simulink model "modelo_ARX"  (R2015a)
settings: Solver=ode45  StartTime=0.0  StopTime=200  RelTol=1e-3
values from neighbouring files (symbols this model uses):
  lambda = 1    [generar_prbs.m]    (also in parametros_ident.m = 0.995)
undefined symbols (not defined in the file or in its folder): sigbuilder_block
settings Model: Creator=u_labelectro  LastModifiedBy=Luis
settings DebuggingCC: UnderspecifiedInitializationDetection=Classic  MergeDetectMultiDrivingBlocksExec=none  SolverPrmCheckMsg=warning  StateNameClashWarn=warning

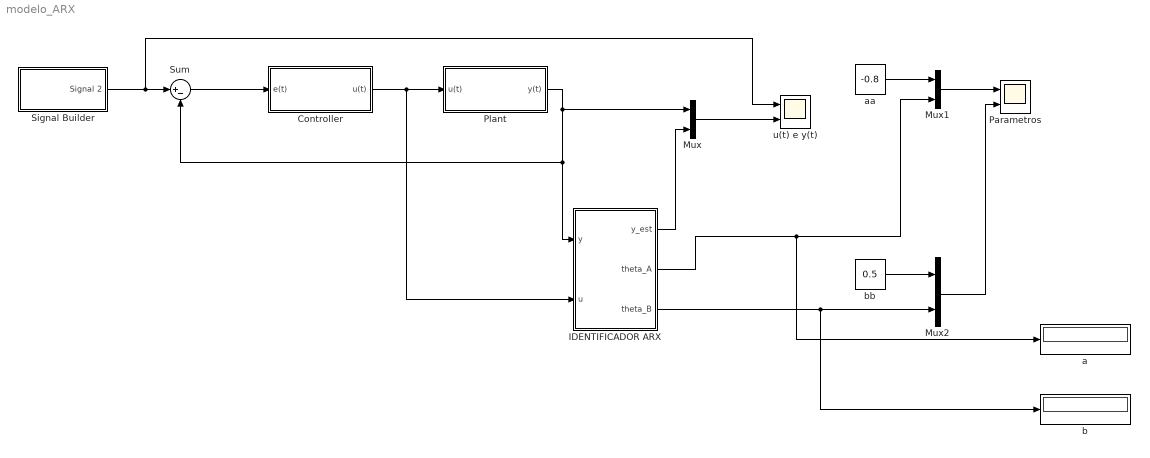
== system modelo_ARX ==
  Controller : Subsystem
  IDENTIFICADOR ARX : Subsystem
  Mux : Mux  Inputs=2
  Mux1 : Mux  Inputs=2
  Mux2 : Mux  Inputs=2
  Parametros : Scope  NumInputPorts=2
      settings: YMin=-5~-5  YMax=5~5
  Plant : Subsystem
  Signal Builder : Subsystem  Tag=STV Subsys  LoadFcn=sigbuilder_block('load',[6 28.5 1068 583.5 ]);  StartFcn=sigbuilder_block('start');  StopFcn=sigbuilder_block('stop');  ClipboardFcn=sigbuilder_block('clipboard');  mask(Sigbuilder block){}
      mask help: Simulink:masks:SigbuilderBlock_MD
      mask init:
      | if ~strcmp(get_param(bdroot(gcbh),'SimulationStatus'),'stopped') tuvar = sigbuilder_block('maskInit'); end
      settings: CopyFcn=sigbuilder_block('copy');  DeleteFcn=sigbuilder_block('delete');  ModelCloseFcn=sigbuilder_block('modelClose');  PreSaveFcn=sigbuilder_block('preSave');  PauseFcn=sigbuilder_block('pause');  ContinueFcn=sigbuilder_block('continue');  NameChangeFcn=sigbuilder_block('namechange');  OpenFcn=sigbuilder_block('open',[6 28.5 1068 583.5 ]);  CloseFcn=sigbuilder_block('close');
      mask Display: plot(0, 0, 100, 100,[2, 2, 32, 32, 2], [68, 8, 8, 68, 68],[32, 2], [38, 38], [32, 19, 2],[53, 60, 44], [32, 17, 17, 2],[16, 16, 31, 31]);txt = getActiveGroup(gcbh);text(2, 100, txt,'verticalAlignment', 'top');
  Sum : Sum  Inputs=|+-
  a : Display
  aa : Constant  Value=-0.8
  b : Display
  bb : Constant  Value=0.5
  u(t) e y(t) : Scope  NumInputPorts=2
      settings: YMin=-5~-5  YMax=5~5  SaveName=ScopeData2
  wires:
  Signal Builder/1(Signal 2) -> u(t) e y(t)/1, Sum/1
  Sum/1 -> Controller/1(e(t))
  Controller/1(u(t)) -> IDENTIFICADOR ARX/2(u), Plant/1(u(t))
  Plant/1(y(t)) -> Mux/1, Sum/2, IDENTIFICADOR ARX/1(y)
  IDENTIFICADOR ARX/1(y_est) -> Mux/2
  Mux/1 -> u(t) e y(t)/2
  aa/1 -> Mux1/1
  IDENTIFICADOR ARX/2(theta_A) -> a/1, Mux1/2
  bb/1 -> Mux2/1
  IDENTIFICADOR ARX/3(theta_B) -> b/1, Mux2/2
  Mux1/1 -> Parametros/1
  Mux2/1 -> Parametros/2

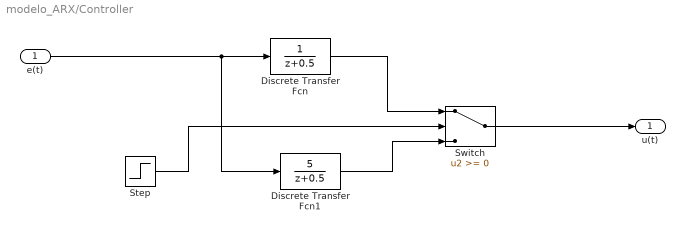
== system modelo_ARX/Controller ==
  e(t) : Inport
  Discrete Transfer Fcn : DiscreteTransferFcn  SampleTime=0.01
  Discrete Transfer Fcn1 : DiscreteTransferFcn  Numerator=[5]  SampleTime=0.01
  Step : Step  Time=50  SampleTime=0
  Switch : Switch
  u(t) : Outport
  wires:
  Step/1 -> Switch/2
  Discrete Transfer Fcn1/1 -> Switch/3
  Discrete Transfer Fcn/1 -> Switch/1
  e(t)/1 -> Discrete Transfer Fcn1/1, Discrete Transfer Fcn/1
  Switch/1 -> u(t)/1

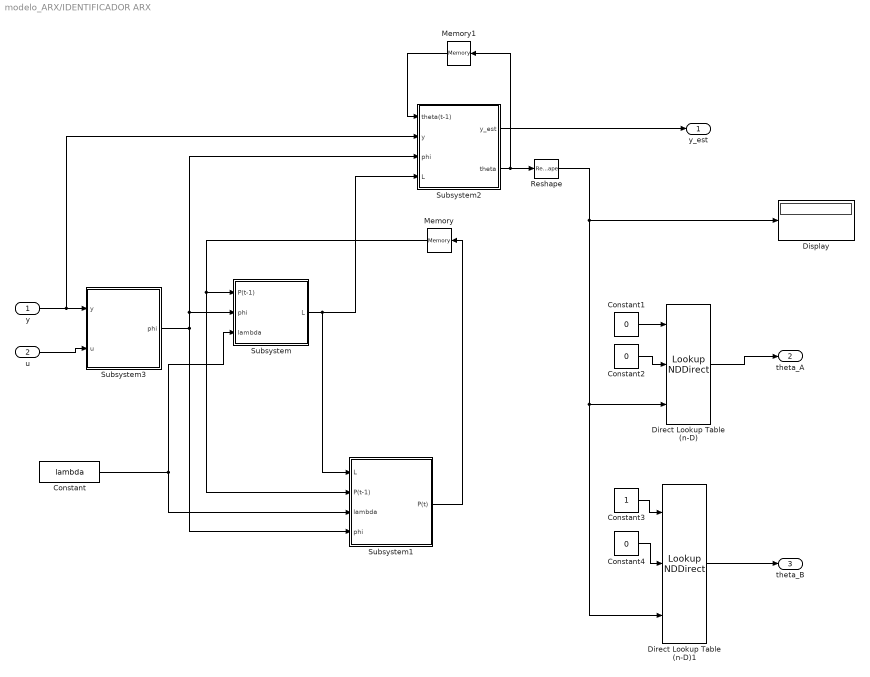
== system modelo_ARX/IDENTIFICADOR ARX ==
  y : Inport
  u : Inport  Port=2
  Constant : Constant  Value=lambda
  Constant1 : Constant  Value=0
  Constant2 : Constant  Value=0
  Constant3 : Constant
  Constant4 : Constant  Value=0
  Direct Lookup Table (n-D) : LookupNDDirect  TableIsInput=on  Table=[4 5 ;16 19 ]  DiagnosticForOutOfRangeInput=Error
  Direct Lookup Table (n-D)1 : LookupNDDirect  TableIsInput=on  Table=[4 5 ;16 19 ]  DiagnosticForOutOfRangeInput=Error
  Display : Display
  Memory : Memory  X0=1e6*eye(2)
  Memory1 : Memory
  Reshape : Reshape  OutputDimensionality=Column vector (2-D)
  Subsystem : Subsystem
  Subsystem1 : Subsystem
  Subsystem2 : Subsystem
  Subsystem3 : Subsystem
  y_est : Outport
  theta_A : Outport  Port=2
  theta_B : Outport  Port=3
  wires:
  y/1 -> Subsystem2/2(y), Subsystem3/1(y)
  Subsystem3/1(phi) -> Subsystem1/4(phi), Subsystem2/3(phi), Subsystem/2(phi)
  Subsystem/1(L) -> Subsystem1/1(L), Subsystem2/4(L)
  u/1 -> Subsystem3/2(u)
  Constant/1 -> Subsystem1/3(lambda), Subsystem/3(lambda)
  Subsystem1/1(P(t)) -> Memory/1
  Memory/1 -> Subsystem1/2(P(t-1)), Subsystem/1(P(t-1))
  Subsystem2/1(y_est) -> y_est/1
  Subsystem2/2(theta) -> Reshape/1, Memory1/1
  Memory1/1 -> Subsystem2/1(theta(t-1))
  Constant4/1 -> Direct Lookup Table (n-D)1/2
  Constant3/1 -> Direct Lookup Table (n-D)1/1
  Constant2/1 -> Direct Lookup Table (n-D)/2
  Constant1/1 -> Direct Lookup Table (n-D)/1
  Reshape/1 -> Direct Lookup Table (n-D)1/3, Direct Lookup Table (n-D)/3, Display/1
  Direct Lookup Table (n-D)/1 -> theta_A/1
  Direct Lookup Table (n-D)1/1 -> theta_B/1

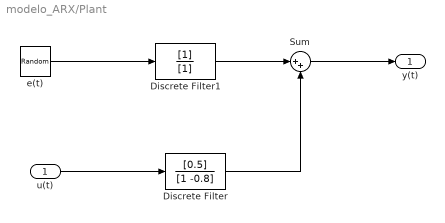
== system modelo_ARX/Plant ==
  u(t) : Inport
  Discrete Filter : DiscreteFilter  Numerator=[0.5]  Denominator=[1 -0.8]  SampleTime=0.01
  Discrete Filter1 : DiscreteFilter  Denominator=[1]
  Sum : Sum  Inputs=|++
  e(t) : RandomNumber  Variance=0.001  SampleTime=0.1
  y(t) : Outport
  wires:
  Discrete Filter/1 -> Sum/2
  Discrete Filter1/1 -> Sum/1
  Sum/1 -> y(t)/1
  u(t)/1 -> Discrete Filter/1
  e(t)/1 -> Discrete Filter1/1

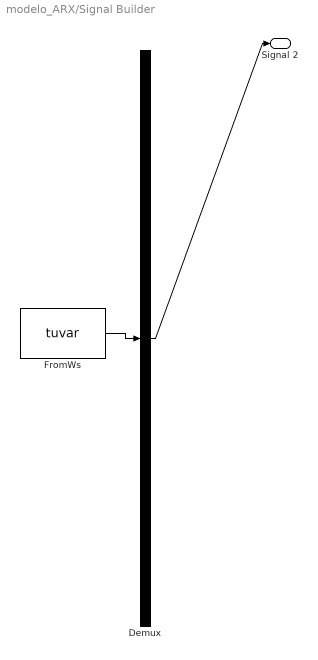
== system modelo_ARX/Signal Builder ==
  Demux : Demux  Tag=STV Demux  Outputs=1
  FromWs : FromWorkspace  Tag=STV FromWs  VariableName=tuvar  SampleTime=0
      SigBuilderData=|
      | common.afterFinalStr = 'Extrapolate'
      | common.sampleTime = 0
      | dataSet.timeRange = [0 100]
      | dataSet.name = 'Group 1'
      | sbobj.Groups.Name = 'Group 1'
      | sbobj.Groups.Signals.Name = 'Signal 2'
      | sbobj.Groups.Signals.XData = [0 10 10 20 100]
      | sbobj.Groups.Signals.YData = [0 0.002 0.496 0.5 0.5]
      | sbobj.Groups.TimeRange = [0 100]
  Signal 2 : Outport  Tag=STV Outport
  wires:
  FromWs/1 -> Demux/1
  Demux/1 -> Signal 2/1

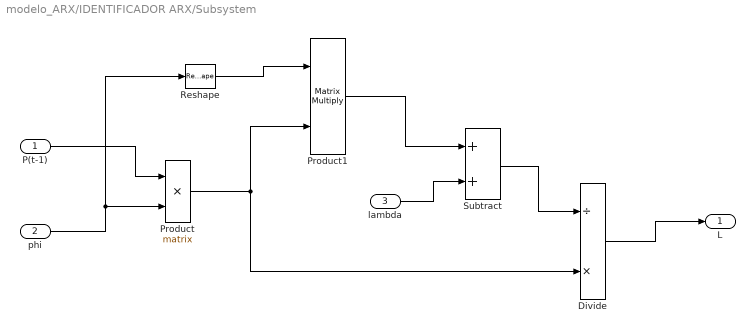
== system modelo_ARX/IDENTIFICADOR ARX/Subsystem ==
  P(t-1) : Inport
  phi : Inport  Port=2
  lambda : Inport  Port=3
  Divide : Product  Inputs=/*
  Product : Product  Multiplication=Matrix(*)
  Product1 : Product  Multiplication=Matrix(*)
  Reshape : Reshape  OutputDimensionality=Row vector (2-D)
  Subtract : Sum
  L : Outport
  wires:
  Divide/1 -> L/1
  Subtract/1 -> Divide/1
  phi/1 -> Reshape/1, Product/2
  Reshape/1 -> Product1/1
  Product1/1 -> Subtract/1
  lambda/1 -> Subtract/2
  Product/1 -> Product1/2, Divide/2
  P(t-1)/1 -> Product/1

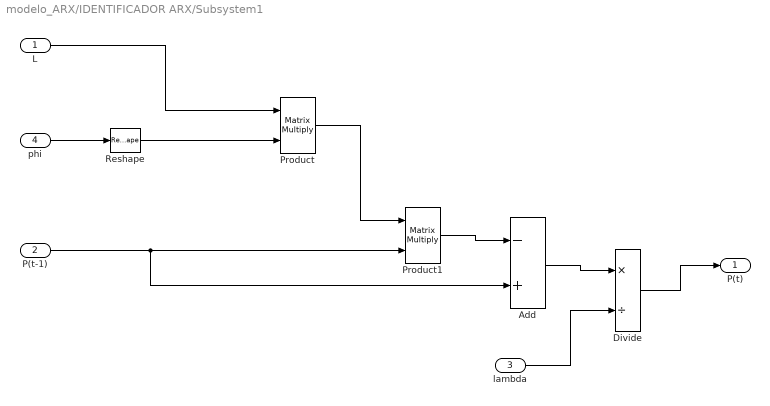
== system modelo_ARX/IDENTIFICADOR ARX/Subsystem1 ==
  L : Inport
  P(t-1) : Inport  Port=2
  lambda : Inport  Port=3
  phi : Inport  Port=4
  Add : Sum  Inputs=-+
  Divide : Product  Inputs=*/
  Product : Product  Multiplication=Matrix(*)
  Product1 : Product  Multiplication=Matrix(*)
  Reshape : Reshape  OutputDimensionality=Row vector (2-D)
  P(t) : Outport
  wires:
  L/1 -> Product/1
  phi/1 -> Reshape/1
  Reshape/1 -> Product/2
  Product/1 -> Product1/1
  P(t-1)/1 -> Add/2, Product1/2
  Product1/1 -> Add/1
  Add/1 -> Divide/1
  Divide/1 -> P(t)/1
  lambda/1 -> Divide/2

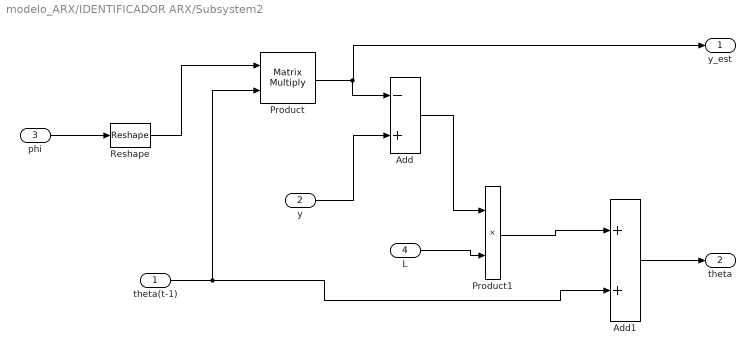
== system modelo_ARX/IDENTIFICADOR ARX/Subsystem2 ==
  theta(t-1) : Inport
  y : Inport  Port=2
  phi : Inport  Port=3
  L : Inport  Port=4
  Add : Sum  Inputs=-+
  Add1 : Sum
  Product : Product  Multiplication=Matrix(*)
  Product1 : Product
  Reshape : Reshape  OutputDimensionality=Row vector (2-D)
  y_est : Outport
  theta : Outport  Port=2
  wires:
  Product/1 -> Add/1, y_est/1
  y/1 -> Add/2
  L/1 -> Product1/2
  Add/1 -> Product1/1
  Product1/1 -> Add1/1
  Add1/1 -> theta/1
  theta(t-1)/1 -> Product/2, Add1/2
  Reshape/1 -> Product/1
  phi/1 -> Reshape/1

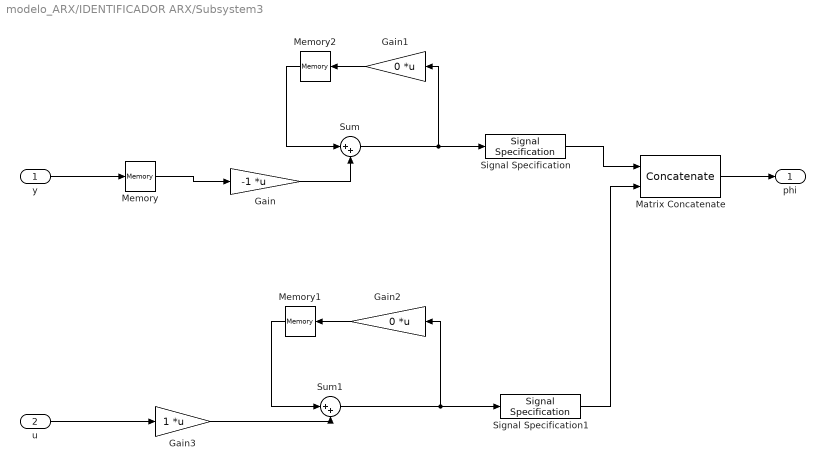
== system modelo_ARX/IDENTIFICADOR ARX/Subsystem3 ==
  y : Inport
  u : Inport  Port=2
  Gain : Gain  Gain=-1  Multiplication=Matrix(K*u)
  Gain1 : Gain  Gain=0  Multiplication=Matrix(K*u)
  Gain2 : Gain  Gain=0  Multiplication=Matrix(K*u)
  Gain3 : Gain  Multiplication=Matrix(K*u)
  Matrix Concatenate : Concatenate  Mode=Multidimensional array
  Memory : Memory
  Memory1 : Memory
  Memory2 : Memory
  Signal Specification : SignalSpecification  Dimensions=[1 1]
  Signal Specification1 : SignalSpecification  Dimensions=[1 1]
  Sum : Sum  Inputs=|++
  Sum1 : Sum  Inputs=|++
  phi : Outport
  wires:
  Sum/1 -> Gain1/1, Signal Specification/1
  Gain1/1 -> Memory2/1
  Memory2/1 -> Sum/1
  Gain/1 -> Sum/2
  Memory/1 -> Gain/1
  y/1 -> Memory/1
  Gain2/1 -> Memory1/1
  u/1 -> Gain3/1
  Gain3/1 -> Sum1/2
  Memory1/1 -> Sum1/1
  Sum1/1 -> Signal Specification1/1, Gain2/1
  Signal Specification/1 -> Matrix Concatenate/1
  Signal Specification1/1 -> Matrix Concatenate/2
  Matrix Concatenate/1 -> phi/1
